simulink model "Speed_PI"  (R2014b)
settings: Solver=ode45  StartTime=0.0  StopTime=0.1  RelTol=1e-3
undefined symbols (not defined in the file): Ba, flux, Init, Kid, Kiq, Kiw, Kpd, Kpq, Kpw, Ld, LowerLimit, Lq, Ts, UpperLimit
settings Model: Creator=Lei  LastModifiedBy=Lei

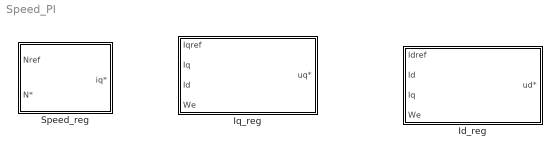
== system Speed_PI ==
  Id_reg : Subsystem
  Iq_reg : Subsystem
  Speed_reg : Subsystem

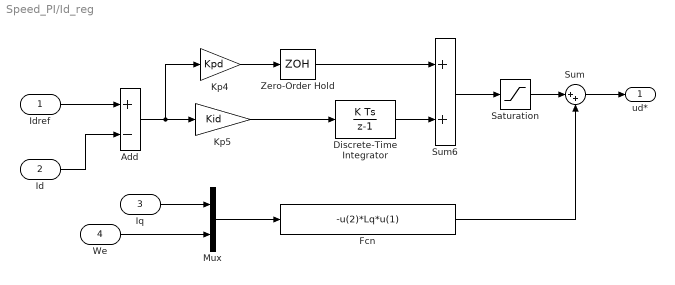
== system Speed_PI/Id_reg ==
  Idref : Inport
  Id : Inport  Port=2
  Iq : Inport  Port=3
  We : Inport  Port=4
  Add : Sum  Inputs=+-
  Discrete-Time Integrator : DiscreteIntegrator  InitialCondition=Init  SampleTime=Ts  UpperSaturationLimit=UpperLimit  LowerSaturationLimit=LowerLimit
  Fcn : Fcn  Expr=-u(2)*Lq*u(1)
  Kp4 : Gain  Gain=Kpd  SampleTime=Ts  SaturateOnIntegerOverflow=on  OutDataTypeStr=Inherit: Same as input  ParamDataTypeStr=Inherit: Same as input
  Kp5 : Gain  Gain=Kid  SampleTime=Ts  SaturateOnIntegerOverflow=on  OutDataTypeStr=Inherit: Same as input  ParamDataTypeStr=Inherit: Same as input
  Mux : Mux  Inputs=2
  Saturation : Saturate
  Sum : Sum  Inputs=|++
  Sum6 : Sum  SampleTime=Ts  SaturateOnIntegerOverflow=on  InputSameDT=on  OutDataTypeStr=Inherit: Same as first input
  Zero-Order Hold : ZeroOrderHold  SampleTime=Ts
  ud* : Outport
  wires:
  Fcn/1 -> Sum/2
  We/1 -> Mux/2
  Iq/1 -> Mux/1
  Mux/1 -> Fcn/1
  Sum/1 -> ud*/1
  Saturation/1 -> Sum/1
  Idref/1 -> Add/1
  Id/1 -> Add/2
  Sum6/1 -> Saturation/1
  Zero-Order Hold/1 -> Sum6/1
  Discrete-Time Integrator/1 -> Sum6/2
  Kp4/1 -> Zero-Order Hold/1
  Kp5/1 -> Discrete-Time Integrator/1
  Add/1 -> Kp5/1, Kp4/1

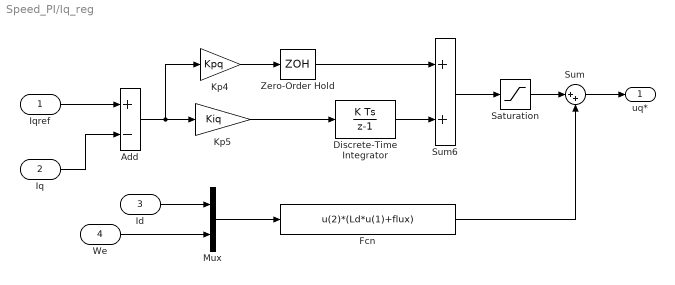
== system Speed_PI/Iq_reg ==
  Iqref : Inport
  Iq : Inport  Port=2
  Id : Inport  Port=3
  We : Inport  Port=4
  Add : Sum  Inputs=+-
  Discrete-Time Integrator : DiscreteIntegrator  InitialCondition=Init  SampleTime=Ts  UpperSaturationLimit=UpperLimit  LowerSaturationLimit=LowerLimit
  Fcn : Fcn  Expr=u(2)*(Ld*u(1)+flux)
  Kp4 : Gain  Gain=Kpq  SampleTime=Ts  SaturateOnIntegerOverflow=on  OutDataTypeStr=Inherit: Same as input  ParamDataTypeStr=Inherit: Same as input
  Kp5 : Gain  Gain=Kiq  SampleTime=Ts  SaturateOnIntegerOverflow=on  OutDataTypeStr=Inherit: Same as input  ParamDataTypeStr=Inherit: Same as input
  Mux : Mux  Inputs=2
  Saturation : Saturate
  Sum : Sum  Inputs=|++
  Sum6 : Sum  SampleTime=Ts  SaturateOnIntegerOverflow=on  InputSameDT=on  OutDataTypeStr=Inherit: Same as first input
  Zero-Order Hold : ZeroOrderHold  SampleTime=Ts
  uq* : Outport
  wires:
  Add/1 -> Kp4/1, Kp5/1
  Kp5/1 -> Discrete-Time Integrator/1
  Kp4/1 -> Zero-Order Hold/1
  Discrete-Time Integrator/1 -> Sum6/2
  Zero-Order Hold/1 -> Sum6/1
  Sum6/1 -> Saturation/1
  Iq/1 -> Add/2
  Iqref/1 -> Add/1
  Saturation/1 -> Sum/1
  Sum/1 -> uq*/1
  Mux/1 -> Fcn/1
  Id/1 -> Mux/1
  We/1 -> Mux/2
  Fcn/1 -> Sum/2

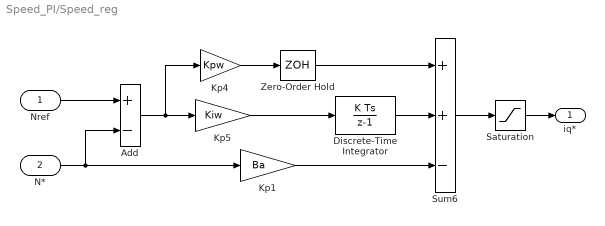
== system Speed_PI/Speed_reg ==
  Nref : Inport
  N* : Inport  Port=2
  Add : Sum  Inputs=+-
  Discrete-Time Integrator : DiscreteIntegrator  InitialCondition=Init  SampleTime=Ts  UpperSaturationLimit=UpperLimit  LowerSaturationLimit=LowerLimit
  Kp1 : Gain  Gain=Ba  SampleTime=Ts  SaturateOnIntegerOverflow=on  OutDataTypeStr=Inherit: Same as input  ParamDataTypeStr=Inherit: Same as input
  Kp4 : Gain  Gain=Kpw  SampleTime=Ts  SaturateOnIntegerOverflow=on  OutDataTypeStr=Inherit: Same as input  ParamDataTypeStr=Inherit: Same as input
  Kp5 : Gain  Gain=Kiw  SampleTime=Ts  SaturateOnIntegerOverflow=on  OutDataTypeStr=Inherit: Same as input  ParamDataTypeStr=Inherit: Same as input
  Saturation : Saturate
  Sum6 : Sum  Inputs=++-  SampleTime=Ts  SaturateOnIntegerOverflow=on  InputSameDT=on  OutDataTypeStr=Inherit: Same as first input
  Zero-Order Hold : ZeroOrderHold  SampleTime=Ts
  iq* : Outport
  wires:
  Nref/1 -> Add/1
  N*/1 -> Kp1/1, Add/2
  Sum6/1 -> Saturation/1
  Zero-Order Hold/1 -> Sum6/1
  Discrete-Time Integrator/1 -> Sum6/2
  Kp4/1 -> Zero-Order Hold/1
  Kp5/1 -> Discrete-Time Integrator/1
  Add/1 -> Kp5/1, Kp4/1
  Saturation/1 -> iq*/1
  Kp1/1 -> Sum6/3
